simulink model "AMR_MoboticControlUnit_24a"  (R2024a)
settings: Solver=FixedStepAuto  StartTime=0.0  StopTime=inf  FixedStep=1e-3  RelTol=1e-3
model workspace (MAT data in the model file):
  mdlWSDbList = "C:\Users\matlab.cut\Desktop\AMR\canbus_files\tramontina_database_mobotic.dbc"
  mobotic_mechanical_offset = -30
libraries: hdlsllib x4, slrealtimeutilitieslib x1
settings Model: Creator=matlab.cut  LastModifiedBy=matlab.cut
settings SolverCC: ConcurrentTasks=on  PositivePriorityOrder=on  AutoInsertRateTranBlk=on
settings OptimizationCC: BlockReduction=off  DefaultParameterBehavior=Inlined  OptimizeBlockIOStorage=off
settings DebuggingCC: TasksWithSamePriorityMsg=none
settings HardwareCC: ProdBitPerLong=64  ProdLongLongMode=on  ProdHWDeviceType=Intel->x86-64 (Linux 64)
settings ModelReferenceCC: ModelReferenceNumInstancesAllowed=Single
settings SFSimCC: MATLABDynamicMemAlloc=off
settings RTWCC: Description=Speedgoat Real-Time Target Machine  SystemTargetFile=speedgoat.tlc  TemplateMakefile=slrealtime_default_tmf  Toolchain=Simulink Real-Time Toolchain  BuildConfiguration=Faster Runs  CodeExecutionProfiling=on  TargetLang=C++  GPUComputeCapability=3.5
settings CodeAppCC: MaxIdLength=127
settings SimulinkRealTimeTargetCC: InstructionSetFMA=off  LogToMDFFile=off

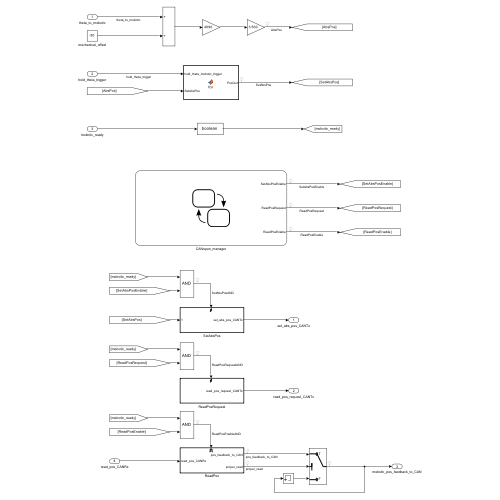
[thumbnail: Simulink's stored preview of the top-level diagram]
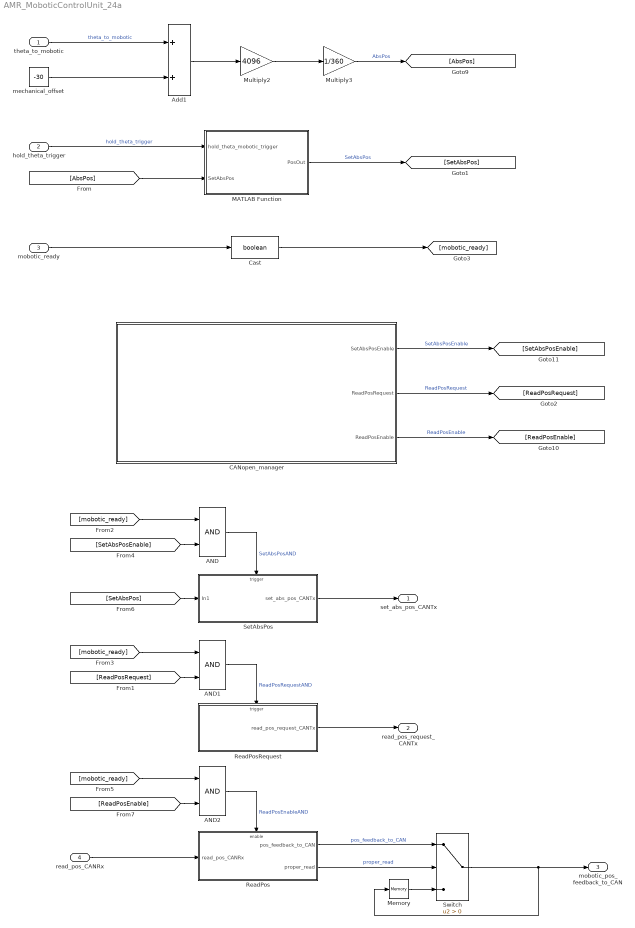
== system AMR_MoboticControlUnit_24a ==
  theta_to_mobotic : Inport
  hold_theta_trigger : Inport  Port=2  OutDataTypeStr=boolean
  mobotic_ready : Inport  Port=3  OutDataTypeStr=boolean
  read_pos_CANRx : Inport  Port=4
  AND : Logic  AllPortsSameDT=off  OutDataTypeStr=boolean
  AND1 : Logic  AllPortsSameDT=off  OutDataTypeStr=boolean
  AND2 : Logic  AllPortsSameDT=off  OutDataTypeStr=boolean
  Add1 : Sum
  CANopen_manager : Stateflow chart  TreatAsAtomicUnit=on
  Cast : DataTypeConversion  OutDataTypeStr=boolean  SaturateOnIntegerOverflow=off  RndMeth=Floor
  MATLAB Function : MATLAB Function  TreatAsAtomicUnit=on
  Memory : Memory
  Multiply2 : Gain  Gain=4096
  Multiply3 : Gain  Gain=1/360
  ReadPos : Subsystem  TreatAsAtomicUnit=on
  ReadPosRequest : Subsystem  TreatAsAtomicUnit=on
  SetAbsPos : Subsystem  TreatAsAtomicUnit=on
  Switch : Switch  Criteria=u2 > Threshold  SaturateOnIntegerOverflow=off  InputSameDT=off
  mechanical_offset : Constant  Value=-30
  set_abs_pos_CANTx : Outport
  read_pos_request_CANTx : Outport  Port=2
  mobotic_pos_feedback_to_CAN : Outport  Port=3
  wires:
  Multiply3/1 -> [AbsPos]  "AbsPos"
  CANopen_manager/3(ReadPosEnable) -> [ReadPosEnable]  "ReadPosEnable"
  mechanical_offset/1 -> Add1/2
  Add1/1 -> Multiply2/1
  [SetAbsPos] -> SetAbsPos/1(In1)
  Multiply2/1 -> Multiply3/1
  CANopen_manager/1(SetAbsPosEnable) -> [SetAbsPosEnable]  "SetAbsPosEnable"
  theta_to_mobotic/1 -> Add1/1  "theta_to_mobotic"
  [AbsPos] -> MATLAB Function/2(SetAbsPos)
  MATLAB Function/1(PosOut) -> [SetAbsPos]  "SetAbsPos"
  hold_theta_trigger/1 -> MATLAB Function/1(hold_theta_mobotic_trigger)  "hold_theta_trigger"
  CANopen_manager/2(ReadPosRequest) -> [ReadPosRequest]  "ReadPosRequest"
  ReadPos/2(proper_read) -> Switch/2  "proper_read"
  Memory/1 -> Switch/3
  ReadPos/1(pos_feedback_to_CAN) -> Switch/1  "pos_feedback_to_CAN"
  Switch/1 -> mobotic_pos_feedback_to_CAN/1, Memory/1
  mobotic_ready/1 -> Cast/1
  [SetAbsPosEnable] -> AND/2
  [mobotic_ready] -> AND/1
  [mobotic_ready] -> AND1/1
  [ReadPosRequest] -> AND1/2
  [mobotic_ready] -> AND2/1
  [ReadPosEnable] -> AND2/2
  Cast/1 -> [mobotic_ready]
  SetAbsPos/1(set_abs_pos_CANTx) -> set_abs_pos_CANTx/1
  ReadPosRequest/1(read_pos_request_CANTx) -> read_pos_request_CANTx/1
  read_pos_CANRx/1 -> ReadPos/1(read_pos_CANRx)
  AND2/1 -> ReadPos/Enable  "ReadPosEnableAND"
  AND/1 -> SetAbsPos/Trigger  "SetAbsPosAND"
  AND1/1 -> ReadPosRequest/Trigger  "ReadPosRequestAND"

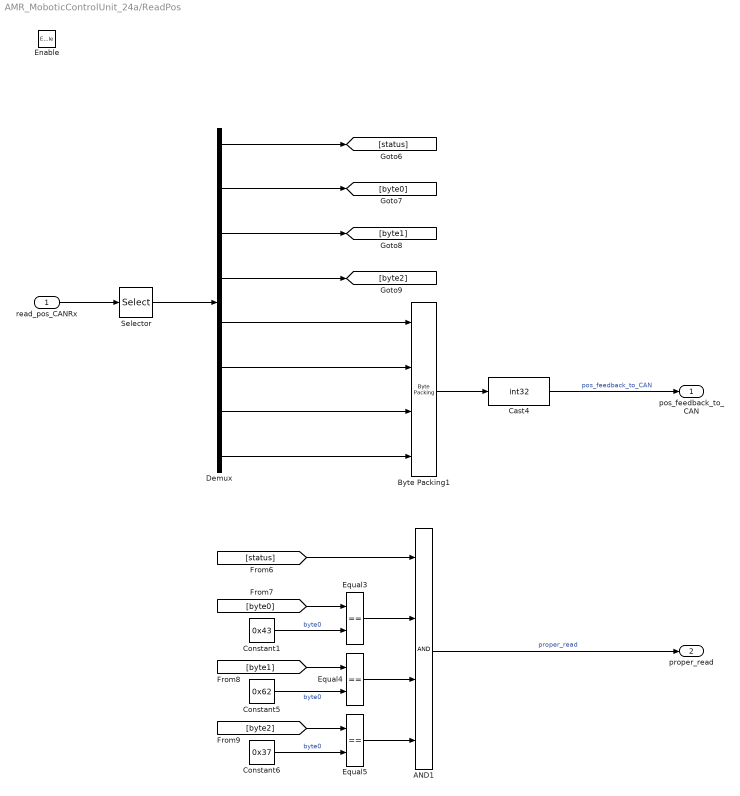
== system AMR_MoboticControlUnit_24a/ReadPos ==
  read_pos_CANRx : Inport
  Enable : EnablePort
  AND1 : Logic  Inputs=4  AllPortsSameDT=off  OutDataTypeStr=boolean
  Byte Packing1 : slrealtimeutilitieslib/Byte Packing  MaskPackedDataType=int32  MaskUnpackedDataTypes={'uint8','uint8','uint8','uint8'}  MaskAlignment=1
  Cast4 : DataTypeConversion  OutDataTypeStr=int32  SaturateOnIntegerOverflow=off  RndMeth=Floor
  Constant1 : Constant  Value=0x43
  Constant5 : Constant  Value=0x62
  Constant6 : Constant  Value=0x37
  Demux : Demux  Outputs=8
  Equal3 : RelationalOperator  Operator===  OutDataTypeStr=boolean  RndMeth=Simplest  InputSameDT=off
  Equal4 : RelationalOperator  Operator===  OutDataTypeStr=boolean  RndMeth=Simplest  InputSameDT=off
  Equal5 : RelationalOperator  Operator===  OutDataTypeStr=boolean  RndMeth=Simplest  InputSameDT=off
  Selector : Selector  IndexMode=Zero-based  InputPortWidth=9  IndexOptions=Index vector (dialog)  Indices=[0:3, 5:8]  OutputSizes=1
  pos_feedback_to_CAN : Outport  InitialOutput=0
  proper_read : Outport  Port=2  InitialOutput=0
  wires:
  Equal5/1 -> AND1/4
  [byte0] -> Equal3/1
  Constant5/1 -> Equal4/2  "byte0"
  [byte1] -> Equal4/1
  [byte2] -> Equal5/1
  Demux/4 -> [byte2]
  [status] -> AND1/1
  Demux/2 -> [byte0]
  Demux/1 -> [status]
  Equal4/1 -> AND1/3
  AND1/1 -> proper_read/1  "proper_read"
  Equal3/1 -> AND1/2
  Byte Packing1/1 -> Cast4/1
  Constant6/1 -> Equal5/2  "byte0"
  Demux/3 -> [byte1]
  Constant1/1 -> Equal3/2  "byte0"
  Cast4/1 -> pos_feedback_to_CAN/1  "pos_feedback_to_CAN"
  Demux/6 -> Byte Packing1/2
  Demux/5 -> Byte Packing1/1
  Demux/7 -> Byte Packing1/3
  Demux/8 -> Byte Packing1/4
  read_pos_CANRx/1 -> Selector/1
  Selector/1 -> Demux/1

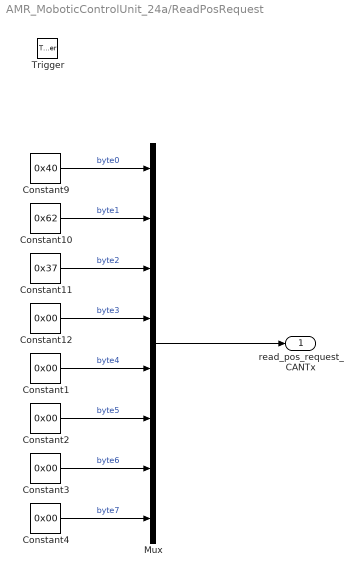
== system AMR_MoboticControlUnit_24a/ReadPosRequest ==
  Trigger : TriggerPort  VariantControl=(inherit)  PortDimensions=1
  Constant{1..4,12} (5 alike) : Constant  Value=0x00
  Constant10 : Constant  Value=0x62
  Constant11 : Constant  Value=0x37
  Constant9 : Constant  Value=0x40
  Mux : Mux  Inputs=8
  read_pos_request_CANTx : Outport  OutputWhenDisabled=reset  InitialOutput=0
  wires:
  Constant12/1 -> Mux/4  "byte3"
  Constant1/1 -> Mux/5  "byte4"
  Constant10/1 -> Mux/2  "byte1"
  Constant11/1 -> Mux/3  "byte2"
  Constant9/1 -> Mux/1  "byte0"
  Constant2/1 -> Mux/6  "byte5"
  Constant3/1 -> Mux/7  "byte6"
  Constant4/1 -> Mux/8  "byte7"
  Mux/1 -> read_pos_request_CANTx/1

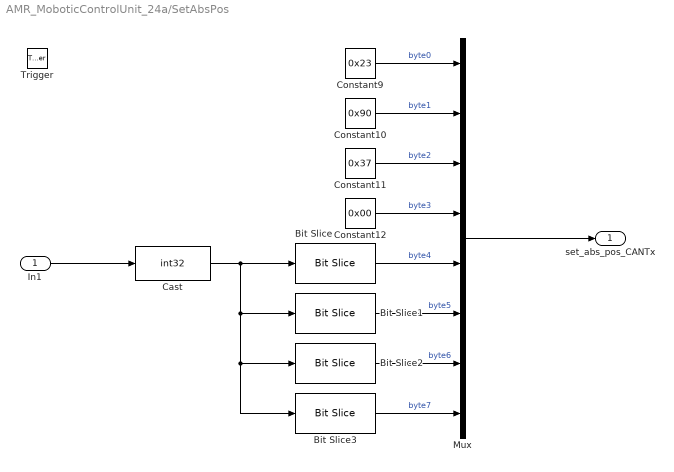
== system AMR_MoboticControlUnit_24a/SetAbsPos ==
  In1 : Inport
  Trigger : TriggerPort  VariantControl=(inherit)  PortDimensions=1
  Bit Slice : hdlsllib/Logic and Bit Operations/Bit Slice  lidx=7  ridx=0
  Bit Slice1 : hdlsllib/Logic and Bit Operations/Bit Slice  lidx=15  ridx=8
  Bit Slice2 : hdlsllib/Logic and Bit Operations/Bit Slice  lidx=23  ridx=16
  Bit Slice3 : hdlsllib/Logic and Bit Operations/Bit Slice  lidx=31  ridx=24
  Cast : DataTypeConversion  OutDataTypeStr=int32  SaturateOnIntegerOverflow=off  RndMeth=Floor
  Constant10 : Constant  Value=0x90
  Constant11 : Constant  Value=0x37
  Constant12 : Constant  Value=0x00
  Constant9 : Constant  Value=0x23
  Mux : Mux  Inputs=8
  set_abs_pos_CANTx : Outport  OutputWhenDisabled=reset  InitialOutput=0
  wires:
  Constant9/1 -> Mux/1  "byte0"
  Constant12/1 -> Mux/4  "byte3"
  Constant11/1 -> Mux/3  "byte2"
  Constant10/1 -> Mux/2  "byte1"
  Bit Slice/1 -> Mux/5  "byte4"
  Bit Slice1/1 -> Mux/6  "byte5"
  Bit Slice2/1 -> Mux/7  "byte6"
  Bit Slice3/1 -> Mux/8  "byte7"
  In1/1 -> Cast/1
  Cast/1 -> Bit Slice3/1, Bit Slice2/1, Bit Slice1/1, Bit Slice/1
  Mux/1 -> set_abs_pos_CANTx/1

== matlab function AMR_MoboticControlUnit_24a/MATLAB Function ==
  data: hold_theta_mobotic_trigger input; SetAbsPos input; PosOut output
function PosOut = fcn(hold_theta_mobotic_trigger, SetAbsPos)
% Function to select output depending on hold_theta_mobotic On/Off status

persistent PosAux  % Declaring PosAux as persistent to retain its value between function calls

if isempty(PosAux)  % Initialize PosAux if it's empty
    PosAux = 0;
end

if hold_theta_mobotic_trigger == 1
    PosOut = SetAbsPos;
    PosAux = PosOut;
else
    PosOut = PosAux;
end

== stateflow chart AMR_MoboticControlUnit_24a/CANopen_manager ==
  state SetAbsPos
    % set flag to run SetAbsPos_Subsystem
    entry:
    SetAbsPosEnable = 1;
    ReadPosRequest = 0;
    ReadPosEnable = 0;
    exit:
    SetAbsPosEnable = 0;
    state=1;
  state ReadPosRequest
    entry:
    SetAbsPosEnable = 0;
    ReadPosRequest = 1;
    ReadPosEnable = 0;
    exit:
    ReadPosRequest=0;
    state=2;
  state ReadPosFeedback
    entry:
    SetAbsPosEnable = 0;
    ReadPosRequest = 0;
    ReadPosEnable = 1;
    exit:
    ReadPosEnable=0;
    state=3;
  (default) -> SetAbsPos : {SetAbsPosEnable=0}
  (junction 29) -> SetAbsPos
  ReadPosFeedback -> (junction 29) : after(5,msec)
  SetAbsPos -> ReadPosRequest : after(10,msec)
  ReadPosRequest -> ReadPosFeedback : after(5,msec)
  data: SetAbsPosEnable output; ReadPosRequest output; ReadPosEnable output; state local
